simulink model "modell"  (R2013a)
settings: Solver=ode45  SolverMode=SingleTasking  StartTime=0.0  StopTime=10.0  RelTol=1e-3
values from neighbouring files (symbols this model uses):
  A = [0 1 0 0; d3 0 0 0;0 0 0 1; c3 0 0 0]    [startModell.m]
  B = [0 ; d1; 0 ; c1]    [startModell.m]
  beobachterNull = [0;0;0;0]    [startModell.m]
  C = [1 0 0 0; 0 0 1 0]    [startModell.m]
  K = lqr(A,B,Q_ctrl,R_ctrl)    [startModell.m]
  L = lqr(A',C',Q, R)'    [startModell.m]
  Mmax = 1000000    [startModell.m]
  Mmin = -1*Mmax    (= -1000000)    [startModell.m]
  modellNull = [10/180*pi;0;0;0]    [startModell.m]
libraries: simulink x1
settings Model: Creator=wall  LastModifiedBy=timoe
settings DataIOCC: SignalLoggingSaveFormat=ModelDataLogs
settings OptimizationCC: BlockReduction=off  BooleanDataType=off
settings DebuggingCC: SaveWithParameterizedLinksMsg=none  SignalResolutionControl=TryResolveAllWithWarning  SolverPrmCheckMsg=none  MultiTaskDSMMsg=warning  MultiTaskCondExecSysMsg=none  StrictBusMsg=None
settings HardwareCC: TargetUnknown=on
settings RTWCC: IncludeERTFirstTime=on

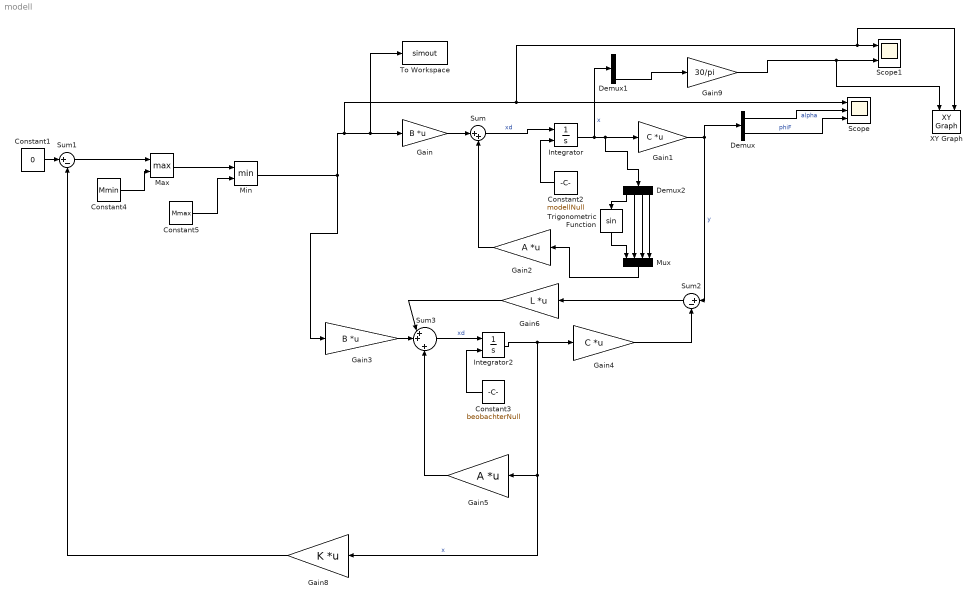
== system modell ==
  Constant1 : Constant  Value=0
  Constant2 : Constant  Value=modellNull
  Constant3 : Constant  Value=beobachterNull
  Constant4 : Constant  Value=Mmin
  Constant5 : Constant  Value=Mmax
  Demux : Demux  Outputs=2
  Demux1 : Demux
  Demux2 : Demux
  Gain : Gain  Gain=B  Multiplication=Matrix(K*u) (u vector)
  Gain1 : Gain  Gain=C  Multiplication=Matrix(K*u) (u vector)
  Gain2 : Gain  Gain=A  Multiplication=Matrix(K*u) (u vector)
  Gain3 : Gain  Gain=B  Multiplication=Matrix(K*u) (u vector)
  Gain4 : Gain  Gain=C  Multiplication=Matrix(K*u) (u vector)
  Gain5 : Gain  Gain=A  Multiplication=Matrix(K*u) (u vector)
  Gain6 : Gain  Gain=L  Multiplication=Matrix(K*u) (u vector)
  Gain8 : Gain  Gain=K  Multiplication=Matrix(K*u) (u vector)
  Gain9 : Gain  Gain=30/pi
  Integrator : Integrator  InitialConditionSource=external
  Integrator2 : Integrator  InitialConditionSource=external
  Max : MinMax  Function=max  Inputs=2
  Min : MinMax  Inputs=2
  Mux : Mux
  Scope : Scope  NumInputPorts=3
      settings: YMin=-1~0.174533~-5  YMax=1~0.174533~5
  Scope1 : Scope  NumInputPorts=2
      settings: YMin=-5~-5  YMax=5~5
  Sum : Sum  Inputs=|++
  Sum1 : Sum  Inputs=|+-
  Sum2 : Sum  Inputs=|+-
  Sum3 : Sum  Inputs=|++|+
  To Workspace : ToWorkspace  VariableName=simout  SampleTime=-1  SaveFormat=Timeseries
  Trigonometric Function : Trigonometry
  XY Graph : simulink/Sinks/XY Graph  xmin=-1  xmax=1  ymin=-1  ymax=1  st=-1
  wires:
  Integrator/1 -> Demux1/1, Demux2/1, Gain1/1  "x"
  Gain1/1 -> Sum2/1, Demux/1  "y"
  Gain2/1 -> Sum/2
  Sum/1 -> Integrator/1  "xd"
  Gain/1 -> Sum/1
  Integrator2/1 -> Gain4/1, Gain8/1, Gain5/1  "x"
  Sum3/1 -> Integrator2/1  "xd"
  Gain4/1 -> Sum2/2
  Sum2/1 -> Gain6/1
  Gain3/1 -> Sum3/2
  Gain5/1 -> Sum3/3
  Gain6/1 -> Sum3/1
  Gain8/1 -> Sum1/2
  Constant1/1 -> Sum1/1
  Constant2/1 -> Integrator/2
  Constant3/1 -> Integrator2/2
  Max/1 -> Min/1
  Constant4/1 -> Max/2
  Sum1/1 -> Max/1
  Constant5/1 -> Min/2
  Min/1 -> XY Graph/2, Scope1/1, Scope/1, To Workspace/1, Gain/1, Gain3/1
  Demux/1 -> Scope/2  "alpha"
  Demux/2 -> Scope/3  "phiF"
  Demux1/4 -> Gain9/1
  Gain9/1 -> XY Graph/1, Scope1/2
  Demux2/1 -> Trigonometric Function/1
  Trigonometric Function/1 -> Mux/1
  Demux2/2 -> Mux/2
  Demux2/3 -> Mux/3
  Demux2/4 -> Mux/4
  Mux/1 -> Gain2/1
